simulink model "TEST_Actuator"  (R2019b)
settings: Solver=ode1  StartTime=0.0  StopTime=110.0  FixedStep=0.004  RelTol=1e-3
libraries: simulink x1, aerolibactuator x1
settings Model: Creator=sl  LastModifiedBy=sl

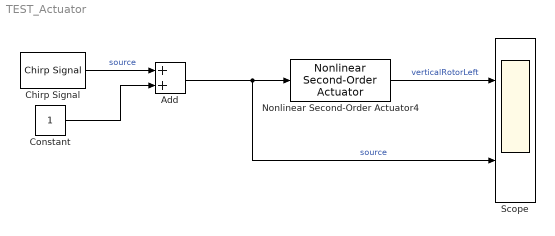
== system TEST_Actuator ==
  Add : Sum
  Chirp Signal : simulink/Sources/Chirp Signal  f1=0.1  T=100  f2=5
  Constant : Constant
  Nonlinear Second-Order Actuator4 : aerolibactuator/Nonlinear Second-Order Actuator  wn_fin=ACTUATOR_SET.verticalRotorLeft.naturalFreq  z_fin=ACTUATOR_SET.verticalRotorLeft.dampingRatio  fin_max=ACTUATOR_SET.verticalRotorLeft.def_max  fin_min=ACTUATOR_SET.verticalRotorLeft.def_min  fin_maxrate=ACTUATOR_SET.verticalRotorLeft.rateLimit  fin_act_0=0  fin_act_vel=0
      settings: SourceProductName=Aerospace Blockset  SourceProductBaseCode=AE
  Scope : Scope  NumInputPorts=2
  wires:
  Add/1 -> Nonlinear Second-Order Actuator4/1, Scope/2  "source"
  Nonlinear Second-Order Actuator4/1 -> Scope/1  "verticalRotorLeft"
  Chirp Signal/1 -> Add/1  "source"
  Constant/1 -> Add/2
